simulink model "IARC_Nonlinear_Sensors"  (R2018a)
settings: Solver=ode1  StartTime=0.0  StopTime=20  FixedStep=T  RelTol=1e-3  EnableMultiTasking=on
undefined symbols (not defined in the file): A_1df, A_2df, alpha3, alpha_rp, alpha_x, alpha_z, an1, an1_v, an2, an3, bn1, bn1_v, bn2, bn3, dc_M_x, delta3, Epsilon3, F, g, Gamma1, Gamma2, Gamma3, Gamma4, gamma4_0, gamma_d_x, gamma_rp_0, gamma_x_0, gamma_z_0, Gammax, I, I_add, I_add_time, Jx, Jy, Jyaw, K, k1, k10, k11, k12, k2, k3, k4, k5, k6, k7, k8, k9, Ky, L, Light, LIMIT_CMD_PITCH, LIMIT_CMD_ROLL, LIMIT_CMD_xy, LIMIT_uCMD_HEIGHT, m, m_add, m_add_time, magnitude, MIL ... (+67)
libraries: simulink x131, simulink_extras x5, UAV_Control x4, aerolibwind2 x1
(part 5 of 6)

== system IARC_Nonlinear_Sensors/ARC Controller/Position Control/Coupling/Warm Up+Sat/Warm Up ==
  u : Inport
  z : Inport  Port=2
  z_des : Inport  Port=3
  " rising " : simulink/Logic and Bit Operations/Compare To Constant  Commented=on  relop=>  const=0  OutDataTypeStr=boolean
  4 : Scope  Commented=on
  6 : Scope  Commented=on
  Compare To Constant1 : simulink/Logic and Bit Operations/Compare To Constant  relop=>=  const=Zg+2/100  OutDataTypeStr=boolean
  Compare To Constant2 : simulink/Logic and Bit Operations/Compare To Constant  relop=>=  const=Zg+2/1000  OutDataTypeStr=boolean
  Data Type Conversion : DataTypeConversion
  Data Type Conversion1 : DataTypeConversion
  Data Type Conversion2 : DataTypeConversion
  InitializationDelay : Subsystem  AncestorBlock=UAV_Control/InitializationDelay  mask(InitializationDelay){t0=t0}
      mask prompts: t0 "Initialization delay:"
      mask help: Applays a delay before passing the first signal.
      mask Help: Applays a delay (t0) before passing the first signal
      mask Display:
      | port_label('input',1,'u','texmode','on')
      | port_label('output',1,'y','texmode','on')
  Is U capable of lifting the quad? : simulink/Logic and Bit Operations/Compare To Constant  relop=>=  const=0.69*m*g  OutDataTypeStr=boolean
  Is the quad commanded to move of the ground? : simulink/Logic and Bit Operations/Compare To Constant  relop=>  const=Zg  OutDataTypeStr=boolean
  Is the quad commanded to move of the ground?1 : simulink/Logic and Bit Operations/Compare To Constant  Commented=on  relop=<=  const=Zg+2/100  OutDataTypeStr=boolean
  Is the quad is commanded to move of the ground?2 : simulink/Logic and Bit Operations/Compare To Constant  relop===  const=Zg  OutDataTypeStr=boolean
  Logical Operator : Logic  AllPortsSameDT=off  OutDataTypeStr=boolean
  Logical Operator1 : Logic  Commented=on  AllPortsSameDT=off  OutDataTypeStr=boolean
  Mux6 : Mux  Commented=on  Inputs=3
  Rate Limiter : RateLimiter  RisingSlewLimit=m*g/2  FallingSlewLimit=-m*g/10  SampleTimeMode=inherited
  Saturation : Saturate  UpperLimit=Sat  LowerLimit=0.001
  Switch : Switch  Criteria=u2 > Threshold  Threshold=0.5
  Triggered Subsystem : Subsystem  TreatAsAtomicUnit=on
  z_ddot : simulink/Discrete/Discrete Derivative  Commented=on  gainval=1.0  ICPrevScaledInput=0.0  InputProcessing=Inherited  OutMin=[]  OutMax=[]  OutDataType=fixdt(1, 16)  OutScaling=2^-10  DoSatur=off
  z_des1 : InportShadow  Port=3
  y : Outport
  Adapt_M : Outport  Port=2
  Adapt_J : Outport  Port=3
  Land : Outport  Port=4
  takeoff2 : Outport  Port=5
  wires:
  u/1 -> Mux6/1, Switch/1, InitializationDelay/1(u)
  InitializationDelay/1(y) -> Rate Limiter/1
  Rate Limiter/1 -> Saturation/1
  Logical Operator/1 -> Data Type Conversion/1
  Data Type Conversion/1 -> Triggered Subsystem/Trigger, Triggered Subsystem/1(" ")
  Triggered Subsystem/1("  ") -> 4/1, Switch/2, Adapt_M/1
  Mux6/1 -> 6/1
  Switch/1 -> Mux6/3, y/1
  z/1 -> Compare To Constant2/1, z_ddot/1, Is the quad commanded to move of the ground?1/1, Compare To Constant1/1
  Compare To Constant1/1 -> Data Type Conversion1/1
  Data Type Conversion1/1 -> Adapt_J/1
  Is U capable of lifting the quad?/1 -> Logical Operator/1
  Is the quad commanded to move of the ground?/1 -> Logical Operator/2
  z_des/1 -> Is the quad commanded to move of the ground?/1
  Saturation/1 -> Mux6/2, Switch/3, Is U capable of lifting the quad?/1
  z_des1/1 -> Is the quad is commanded to move of the ground?2/1
  Is the quad is commanded to move of the ground?2/1 -> Land/1
  Compare To Constant2/1 -> Data Type Conversion2/1
  Data Type Conversion2/1 -> takeoff2/1
  Is the quad commanded to move of the ground?1/1 -> Logical Operator1/1
  z_ddot/1 -> " rising "/1
  " rising "/1 -> Logical Operator1/2
  Logical Operator1/1 -> ?

== system IARC_Nonlinear_Sensors/ARC Controller/Position Control/X control/Adaptation Law_X/  ==
  1 : Scope
  Constant4 : Constant  Value=m
  Divide : Product  Inputs=*/
  Selector : Selector  InputPortWidth=3  IndexOptions=Index vector (dialog)  Indices=1  OutputSizes=1
  Sum : Sum  Inputs=|++
  m_add : Step  Time=m_add_time  After=m_add(1,1)  SampleTime=0
  Out1 : Outport
  wires:
  [Fd] -> Selector/1
  Divide/1 -> 1/1, Out1/1
  Sum/1 -> Divide/2
  Constant4/1 -> Sum/1
  m_add/1 -> Sum/2
  Selector/1 -> Divide/1

== system IARC_Nonlinear_Sensors/ARC Controller/Position Control/X control/Adaptation Law_X/IARC, Physical Model Based Parameter Estimation (69)_X ==
  f(x) : Inport
  Phi : Inport  Port=2
  Adapt : Inport  Port=3
  Adapt1 : InportShadow  Port=3
  Constant2 : Constant  Value=Norm_ON
  Discontinuous_Proj_(49) : Subsystem
  Display : Display  Commented=on
  Divide : Product  Inputs=*/
  Epsilon : Subsystem
  Filter : Subsystem
  Gamma : Subsystem
  Switch1 : Switch  Threshold=0.5
  Theta_hat_dot : Product  Inputs=3  Multiplication=Matrix(*)
  den : Scope  Commented=on
  "epsilon  " : Scope  Commented=on
  gamma : Scope  Commented=on
  theta dot : Scope  Commented=on
  theta hat : Scope  Commented=on
  Theta_hat : Outport
  wires:
  Epsilon/1(Epsilon) -> Theta_hat_dot/3, "epsilon  "/1  "predicted output error"
  Discontinuous_Proj_(49)/1(Theta) -> theta hat/1, Theta_hat/1, Epsilon/3(Theta_hat)
  Filter/1(f(x)_f) -> Epsilon/1(f(x)_f_dot)
  Phi/1 -> Filter/2("Phi ")
  f(x)/1 -> Filter/1(f(x))
  Theta_hat_dot/1 -> Discontinuous_Proj_(49)/1(Theta_dot), theta dot/1
  Constant2/1 -> Switch1/2
  Gamma/1(" gamma") -> Display/1, gamma/1, Switch1/3, Divide/1
  Switch1/1 -> Theta_hat_dot/1
  Divide/1 -> Switch1/1
  Gamma/2(" 1+nu.Phi.G.Phi") -> den/1, Divide/2
  Filter/2(Phi_f) -> Epsilon/2(Phi_f), Gamma/1(Phi_f), Theta_hat_dot/2
  Adapt/1 -> Gamma/2(Adapt)
  Adapt1/1 -> Discontinuous_Proj_(49)/2(Adapt)

== system IARC_Nonlinear_Sensors/ARC Controller/Position Control/X control/Adaptation Law_X/Integral Type Adaptation Law Discontinuous Projection1 ==
  Phi : Inport
  error : Inport  Port=2
  {1..5} (5 alike) : Scope  Commented=on
  Constant : Constant  Value=gamma
  Constant2 : Constant  Value=Adaptation_ON
  Discontinuous Projection : Integrator  InitialCondition=theta0  LimitOutput=on  UpperSaturationLimit=theta_max  LowerSaturationLimit=theta_min
  Discontinuous Projection1 : Integrator  Commented=on  InitialCondition=theta0  UpperSaturationLimit=theta_max  LowerSaturationLimit=theta_min
  Gain : Gain  Commented=on  Gain=PSI
  InitializationDelay : Subsystem  AncestorBlock=UAV_Control/InitializationDelay  mask(InitializationDelay){t0=t1}
      mask prompts: t0 "Initialization delay:"
      mask help: Applays a delay before passing the first signal.
      mask Help: Applays a delay (t0) before passing the first signal
      mask Display:
      | port_label('input',1,'u','texmode','on')
      | port_label('output',1,'y','texmode','on')
  Product1 : Product  Inputs=3  Multiplication=Matrix(*)
  Saturation : Saturate  Commented=on  UpperLimit=theta_max  LowerLimit=theta_min
  Sum : Sum  Commented=on  Inputs=|++
  Sum1 : Sum  Commented=on  Inputs=-|+
  Switch1 : Switch  Criteria=u2 ~= 0
  real : Constant  Value=theta
  theta_est : Outport
  wires:
  Constant/1 -> Product1/1
  error/1 -> 2/1, Product1/3
  real/1 -> Switch1/3
  Constant2/1 -> Switch1/2
  Product1/1 -> InitializationDelay/1(u)
  Phi/1 -> 3/1, Product1/2
  InitializationDelay/1(y) -> Discontinuous Projection/1, 4/1, Sum/1
  Switch1/1 -> theta_est/1
  Sum/1 -> Discontinuous Projection1/1
  Discontinuous Projection1/1 -> Sum1/1, Saturation/1
  Sum1/1 -> Gain/1
  Gain/1 -> Sum/2
  Saturation/1 -> 1/1, Sum1/2
  Discontinuous Projection/1 -> 5/1, Switch1/1

== system IARC_Nonlinear_Sensors/ARC Controller/Position Control/X control/Adaptation Law_X/Subsystem1 ==
  u : Inport
  6 : Scope
  Constant4 : Constant  Value=m
  Divide : Product  Inputs=**
  Sum : Sum  Inputs=|++
  m_add : Step  Time=m_add_time  After=m_add  SampleTime=0
  y : Outport
  wires:
  u/1 -> Divide/1
  m_add/1 -> Sum/2
  Divide/1 -> y/1
  Sum/1 -> Divide/2, 6/1
  Constant4/1 -> Sum/1

== system IARC_Nonlinear_Sensors/ARC Controller/Position Control/Y control/Adaptation Law_Y/  ==
  1 : Scope
  Constant4 : Constant  Value=m
  Divide : Product  Inputs=*/
  Selector : Selector  InputPortWidth=3  IndexOptions=Index vector (dialog)  Indices=1  OutputSizes=1
  Sum : Sum  Inputs=|++
  m_add : Step  Time=m_add_time  After=m_add(1,1)  SampleTime=0
  Out1 : Outport
  wires:
  [Fd] -> Selector/1
  Divide/1 -> 1/1, Out1/1
  Sum/1 -> Divide/2
  Constant4/1 -> Sum/1
  m_add/1 -> Sum/2
  Selector/1 -> Divide/1

== system IARC_Nonlinear_Sensors/ARC Controller/Position Control/Y control/Adaptation Law_Y/IARC, Physical Model Based Parameter Estimation (69)_X ==
  f(x) : Inport
  Phi : Inport  Port=2
  Adapt : Inport  Port=3
  Adapt1 : InportShadow  Port=3
  Constant2 : Constant  Value=Norm_ON
  Discontinuous_Proj_(49) : Subsystem
  Display : Display  Commented=on
  Divide : Product  Inputs=*/
  Epsilon : Subsystem
  Filter : Subsystem
  Gamma : Subsystem
  Switch1 : Switch  Threshold=0.5
  Theta_hat_dot : Product  Inputs=3  Multiplication=Matrix(*)
  "epsilon  " : Scope  Commented=on
  gamma : Scope  Commented=on
  theta dot : Scope  Commented=on
  theta hat : Scope  Commented=on
  Theta_hat : Outport
  wires:
  Epsilon/1(Epsilon) -> Theta_hat_dot/3, "epsilon  "/1  "predicted output error"
  Discontinuous_Proj_(49)/1(Theta) -> theta hat/1, Theta_hat/1, Epsilon/3(Theta_hat)
  Filter/1(f(x)_f) -> Epsilon/1(f(x)_f_dot)
  Phi/1 -> Filter/2("Phi ")
  f(x)/1 -> Filter/1(f(x))
  Theta_hat_dot/1 -> Discontinuous_Proj_(49)/1(Theta_dot), theta dot/1
  Constant2/1 -> Switch1/2
  Gamma/1(" gamma") -> Display/1, gamma/1, Switch1/3, Divide/1
  Switch1/1 -> Theta_hat_dot/1
  Divide/1 -> Switch1/1
  Gamma/2(" 1+nu.Phi.G.Phi") -> Divide/2
  Filter/2(Phi_f) -> Epsilon/2(Phi_f), Gamma/1(Phi_f), Theta_hat_dot/2
  Adapt/1 -> Gamma/2(Adapt)
  Adapt1/1 -> Discontinuous_Proj_(49)/2(Adapt)

== system IARC_Nonlinear_Sensors/ARC Controller/Position Control/Y control/Adaptation Law_Y/Integral Type Adaptation Law Discontinuous Projection1 ==
  Phi : Inport
  error : Inport  Port=2
  {1..5} (5 alike) : Scope  Commented=on
  Constant : Constant  Value=gamma
  Constant2 : Constant  Value=Adaptation_ON
  Discontinuous Projection : Integrator  InitialCondition=theta0  LimitOutput=on  UpperSaturationLimit=theta_max  LowerSaturationLimit=theta_min
  Discontinuous Projection1 : Integrator  Commented=on  InitialCondition=theta0  UpperSaturationLimit=theta_max  LowerSaturationLimit=theta_min
  Gain : Gain  Commented=on  Gain=PSI
  InitializationDelay : Subsystem  AncestorBlock=UAV_Control/InitializationDelay  mask(InitializationDelay){t0=t1}
      mask prompts: t0 "Initialization delay:"
      mask help: Applays a delay before passing the first signal.
      mask Help: Applays a delay (t0) before passing the first signal
      mask Display:
      | port_label('input',1,'u','texmode','on')
      | port_label('output',1,'y','texmode','on')
  Product1 : Product  Inputs=3  Multiplication=Matrix(*)
  Saturation : Saturate  Commented=on  UpperLimit=theta_max  LowerLimit=theta_min
  Sum : Sum  Commented=on  Inputs=|++
  Sum1 : Sum  Commented=on  Inputs=-|+
  Switch1 : Switch  Criteria=u2 ~= 0
  real : Constant  Value=theta
  theta_est : Outport
  wires:
  Constant/1 -> Product1/1
  error/1 -> 2/1, Product1/3
  real/1 -> Switch1/3
  Constant2/1 -> Switch1/2
  Product1/1 -> InitializationDelay/1(u)
  Phi/1 -> 3/1, Product1/2
  InitializationDelay/1(y) -> Discontinuous Projection/1, 4/1, Sum/1
  Switch1/1 -> theta_est/1
  Sum/1 -> Discontinuous Projection1/1
  Discontinuous Projection1/1 -> Sum1/1, Saturation/1
  Sum1/1 -> Gain/1
  Gain/1 -> Sum/2
  Saturation/1 -> 1/1, Sum1/2
  Discontinuous Projection/1 -> 5/1, Switch1/1

== system IARC_Nonlinear_Sensors/ARC Controller/Position Control/Y control/Adaptation Law_Y/Subsystem1 ==
  u : Inport
  6 : Scope
  Constant4 : Constant  Value=m
  Divide : Product  Inputs=**
  Sum : Sum  Inputs=|++
  m_add : Step  Time=m_add_time  After=m_add  SampleTime=0
  y : Outport
  wires:
  u/1 -> Divide/1
  m_add/1 -> Sum/2
  Divide/1 -> y/1
  Sum/1 -> Divide/2, 6/1
  Constant4/1 -> Sum/1

== system IARC_Nonlinear_Sensors/ARC Controller/Position Control/Z control/Estimate theta = K//m/IARC, Physical Model Based Parameter Estimation (69) ==
  y : Inport
  Phi : Inport  Port=2
  Adapt1 : Inport  Port=3
  Adapt2 : InportShadow  Port=3
  Constant2 : Constant  Value=Norm_ON
  Discontinuous_Proj_(49) : Subsystem
  Display : Display  Commented=on
  Divide : Product  Inputs=*/
  Epsilon : Subsystem
  Filter : Subsystem
  Gamma : Subsystem
  Switch1 : Switch  Threshold=0.5
  Theta_hat_dot : Product  Inputs=3  Multiplication=Matrix(*)
  "epsilon  " : Scope  Commented=on
  gamma : Scope  Commented=on
  theta dot : Scope  Commented=on
  theta hat : Scope  Commented=on
  Theta_hat : Outport
  wires:
  Adapt1/1 -> Discontinuous_Proj_(49)/2(Adapt)
  Filter/2(Phi_f) -> Epsilon/2(Phi_f), Gamma/1(Phi_f), Theta_hat_dot/2
  Epsilon/1(Epsilon) -> "epsilon  "/1, Theta_hat_dot/3  "predicted output error"
  Discontinuous_Proj_(49)/1(Theta) -> Theta_hat/1, theta hat/1, Epsilon/3(Theta_hat)
  Filter/1(y_f) -> Epsilon/1(y_f)
  Phi/1 -> Filter/2("Phi ")
  y/1 -> Filter/1(y)
  Theta_hat_dot/1 -> Discontinuous_Proj_(49)/1(Theta_dot), theta dot/1
  Constant2/1 -> Switch1/2
  Gamma/1(" gamma") -> Display/1, gamma/1, Switch1/3, Divide/1
  Switch1/1 -> Theta_hat_dot/1
  Divide/1 -> Switch1/1
  Gamma/2(" 1+nu.Phi.G.Phi") -> Divide/2
  Adapt2/1 -> Gamma/2(Adapt)

== system IARC_Nonlinear_Sensors/ARC Controller/Position Control/Z control/Estimate theta = K//m/Integral Type Adaptation Law Discontinuous Projection ==
  Phi : Inport
  error : Inport  Port=2
  {1..5,11} (6 alike) : Scope  Commented=on
  Constant : Constant  Value=gamma
  Constant2 : Constant  Value=Adaptation_ON
  Discontinuous Projection : Integrator  InitialCondition=theta0  LimitOutput=on  UpperSaturationLimit=theta_max  LowerSaturationLimit=theta_min
  Discontinuous Projection1 : Integrator  Commented=on  InitialCondition=theta0  UpperSaturationLimit=theta_max  LowerSaturationLimit=theta_min
  Gain : Gain  Commented=on  Gain=PSI
  InitializationDelay : Subsystem  AncestorBlock=UAV_Control/InitializationDelay  mask(InitializationDelay){t0=t1}
      mask prompts: t0 "Initialization delay:"
      mask help: Applays a delay before passing the first signal.
      mask Help: Applays a delay (t0) before passing the first signal
      mask Display:
      | port_label('input',1,'u','texmode','on')
      | port_label('output',1,'y','texmode','on')
  Product1 : Product  Inputs=3  Multiplication=Matrix(*)
  Saturation : Saturate  Commented=on  UpperLimit=theta_max  LowerLimit=theta_min
  Sum : Sum  Commented=on  Inputs=|++
  Sum1 : Sum  Commented=on  Inputs=-|+
  Switch1 : Switch  Criteria=u2 ~= 0
  real : Constant  Value=theta
  theta_est : Outport
  wires:
  Constant/1 -> Product1/1
  error/1 -> 2/1, Product1/3
  real/1 -> Switch1/3
  Constant2/1 -> Switch1/2
  Product1/1 -> InitializationDelay/1(u)
  Phi/1 -> 3/1, Product1/2
  InitializationDelay/1(y) -> Discontinuous Projection/1, 4/1, Sum/1, 11/1
  Switch1/1 -> theta_est/1
  Sum/1 -> Discontinuous Projection1/1
  Discontinuous Projection1/1 -> Sum1/1, Saturation/1
  Sum1/1 -> Gain/1
  Gain/1 -> Sum/2
  Saturation/1 -> 1/1, Sum1/2
  Discontinuous Projection/1 -> 5/1, Switch1/1

== system IARC_Nonlinear_Sensors/ARC Controller/Position Control/Z control/Estimate theta = K//m/m ==
  Constant4 : Constant  Value=m
  Gain : Gain  Gain=K
  Math Function : Math  Operator=reciprocal  SaturateOnIntegerOverflow=on
  Step : Step  Time=m_add_time  After=m_add  SampleTime=0
  Sum : Sum  Inputs=|++
  Out1 : Outport
  wires:
  Constant4/1 -> Sum/1
  Step/1 -> Sum/2
  Math Function/1 -> Gain/1
  Gain/1 -> Out1/1
  Sum/1 -> Math Function/1

== system IARC_Nonlinear_Sensors/Sensors and Filters/Data processing/Estimate Position/Signal Conditioning - Sonar/FOH1 ==
  Input : Inport
  Bias : Bias  Bias=-Ts
  Clock : Clock
      settings: DisableCoverage=on
  Digital Clock : DigitalClock  DisableCoverage=on  SampleTime=Ts
  Gain : Gain  DisableCoverage=on  Gain=1/Ts  SaturateOnIntegerOverflow=on  OutDataTypeStr=Inherit: Same as input  ParamDataTypeStr=Inherit: Same as input
  Product : Product  RndMeth=Zero
  Rate Transition : RateTransition
  Rate Transition1 : RateTransition  OutPortSampleTime=T
  Rate Transition3 : RateTransition  OutPortSampleTime=T
  Rate Transition4 : RateTransition  OutPortSampleTime=Ts
  Rate Transition5 : RateTransition  OutPortSampleTime=T
  Scope : Scope
  Scope1 : Scope
  Sum : Sum  DisableCoverage=on  Inputs=|+-  SaturateOnIntegerOverflow=on  InputSameDT=on  OutDataTypeStr=Inherit: Same as first input
  Sum2 : Sum  DisableCoverage=on  Inputs=|+-  SaturateOnIntegerOverflow=on  InputSameDT=on  OutDataTypeStr=Inherit: Same as first input
  Unit Delay : UnitDelay  DisableCoverage=on  SampleTime=Ts
  s : Sum  Inputs=++|  SaturateOnIntegerOverflow=on  InputSameDT=on  OutDataTypeStr=Inherit: Same as first input
  Output : Outport
  wires:
  Rate Transition4/1 -> Unit Delay/1, Sum/1
  Input/1 -> Rate Transition4/1, Rate Transition5/1
  Unit Delay/1 -> Sum/2
  Rate Transition1/1 -> Product/1, Scope1/1
  Product/1 -> s/2
  Rate Transition3/1 -> Product/2, Scope/1
  Sum/1 -> Rate Transition1/1
  Bias/1 -> Sum2/1
  Clock/1 -> Bias/1
  Rate Transition/1 -> Sum2/2
  s/1 -> Output/1
  Rate Transition5/1 -> s/1
  Gain/1 -> Rate Transition3/1
  Digital Clock/1 -> Rate Transition/1
  Sum2/1 -> Gain/1

== system IARC_Nonlinear_Sensors/Sensors and Filters/Data processing/Estimate Position/Signal Conditioning - Sonar/Sampler ==
  In1 : Inport
  Derivative : Derivative
  Digital Clock : DigitalClock  DisableCoverage=on  SampleTime=0.1
  Rate Transition : RateTransition
  Triggered Subsystem : Subsystem  TreatAsAtomicUnit=on
  Out1 : Outport
  wires:
  Derivative/1 -> Triggered Subsystem/Trigger
  Rate Transition/1 -> Derivative/1
  Digital Clock/1 -> Rate Transition/1
  In1/1 -> Triggered Subsystem/1(In1)
  Triggered Subsystem/1(Out1) -> Out1/1

== system IARC_Nonlinear_Sensors/ARC Controller/Attitutde Control/Subsystem/f/d(T)//d(phi)/Subsystem ==
  In1 : Inport
  In2 : Inport  Port=2
  In3 : Inport  Port=3
  In4 : Inport  Port=4
  In5 : Inport  Port=5
  In6 : Inport  Port=6
  In7 : Inport  Port=7
  In8 : Inport  Port=8
  In9 : Inport  Port=9
  Matrix Concatenate : Concatenate  NumInputs=3  Mode=Multidimensional array  ConcatenateDimension=2
  Mux : Mux  Inputs=3
  Mux1 : Mux  Inputs=3
  Mux2 : Mux  Inputs=3
  Reshape : Reshape  OutputDimensionality=Column vector (2-D)
  Reshape1 : Reshape  OutputDimensionality=Column vector (2-D)
  Reshape2 : Reshape  OutputDimensionality=Column vector (2-D)
  Out1 : Outport
  wires:
  Reshape1/1 -> Matrix Concatenate/2
  Mux1/1 -> Reshape1/1
  Reshape/1 -> Matrix Concatenate/1
  Reshape2/1 -> Matrix Concatenate/3
  Matrix Concatenate/1 -> Out1/1
  Mux2/1 -> Reshape2/1
  Mux/1 -> Reshape/1
  In1/1 -> Mux/1
  In2/1 -> Mux/2
  In3/1 -> Mux/3
  In4/1 -> Mux1/1
  In5/1 -> Mux1/2
  In6/1 -> Mux1/3
  In7/1 -> Mux2/1
  In8/1 -> Mux2/2
  In9/1 -> Mux2/3

== system IARC_Nonlinear_Sensors/ARC Controller/Attitutde Control/Subsystem/f/d(T)//d(theta)/Subsystem ==
  In1 : Inport
  In2 : Inport  Port=2
  In3 : Inport  Port=3
  In4 : Inport  Port=4
  In5 : Inport  Port=5
  In6 : Inport  Port=6
  In7 : Inport  Port=7
  In8 : Inport  Port=8
  In9 : Inport  Port=9
  Matrix Concatenate : Concatenate  NumInputs=3  Mode=Multidimensional array  ConcatenateDimension=2
  Mux : Mux  Inputs=3
  Mux1 : Mux  Inputs=3
  Mux2 : Mux  Inputs=3
  Reshape : Reshape  OutputDimensionality=Column vector (2-D)
  Reshape1 : Reshape  OutputDimensionality=Column vector (2-D)
  Reshape2 : Reshape  OutputDimensionality=Column vector (2-D)
  Out1 : Outport
  wires:
  In9/1 -> Mux2/3
  In8/1 -> Mux2/2
  In7/1 -> Mux2/1
  In6/1 -> Mux1/3
  In5/1 -> Mux1/2
  In4/1 -> Mux1/1
  In3/1 -> Mux/3
  In2/1 -> Mux/2
  In1/1 -> Mux/1
  Mux/1 -> Reshape/1
  Mux2/1 -> Reshape2/1
  Matrix Concatenate/1 -> Out1/1
  Reshape2/1 -> Matrix Concatenate/3
  Reshape/1 -> Matrix Concatenate/1
  Mux1/1 -> Reshape1/1
  Reshape1/1 -> Matrix Concatenate/2

== system IARC_Nonlinear_Sensors/ARC Controller/Attitutde Control/Yaw control/Subsystem/IARC, Physical Model Based Parameter Estimation (69)_Yaw/Discontinuous_Proj_(49) ==
  Theta_dot : Inport
  Adapt : Inport  Port=2
  Integrator2 : Integrator  InitialCondition=theta_0  LimitOutput=on  UpperSaturationLimit=theta_max  LowerSaturationLimit=theta_min
  Product : Product
  Saturation : Saturate  UpperLimit=Theta_dot_M  LowerLimit=-Theta_dot_M
  Theta : Outport
  wires:
  Integrator2/1 -> Theta/1
  Product/1 -> Saturation/1
  Saturation/1 -> Integrator2/1
  Adapt/1 -> Product/2
  Theta_dot/1 -> Product/1

== system IARC_Nonlinear_Sensors/ARC Controller/Attitutde Control/Yaw control/Subsystem/IARC, Physical Model Based Parameter Estimation (69)_Yaw/Epsilon ==
  f(x)_f_dot : Inport
  Phi_f : Inport  Port=2
  Theta_hat : Inport  Port=3
  Math Function : Math  Operator=transpose  SaturateOnIntegerOverflow=on
  Mux1 : Mux  Inputs=3
  Product1 : Product  Multiplication=Matrix(*)
  Subtract : Sum  Inputs=+-
  "epsilon  " : Scope
  Epsilon : Outport
  wires:
  f(x)_f_dot/1 -> Mux1/2, Subtract/1  "Yp"
  Product1/1 -> Mux1/3, Subtract/2  "Yp_hat"
  Phi_f/1 -> Math Function/1
  Theta_hat/1 -> Product1/2
  Math Function/1 -> Product1/1
  Subtract/1 -> Mux1/1, Epsilon/1
  Mux1/1 -> "epsilon  "/1

== system IARC_Nonlinear_Sensors/ARC Controller/Attitutde Control/Yaw control/Subsystem/IARC, Physical Model Based Parameter Estimation (69)_Yaw/Filter ==
  f(x) : Inport
  "Phi " : Inport  Port=2
  Demux : Demux  Outputs=2
  Mux1 : Mux  Commented=on  Inputs=2
  Mux2 : Mux  Commented=on  Inputs=2
  Mux3 : Mux  Inputs=2
  filter : TransferFcn  Denominator=[Tau 1]
  "filter " : TransferFcn  Denominator=[Tau 1]
  filter1 : TransferFcn  Denominator=[Tau 1]
  gamma : Scope  Commented=on
  gamma1 : Scope  Commented=on
  f(x)_f : Outport
  Phi_f : Outport  Port=2
  wires:
  "Phi "/1 -> Demux/1
  "filter "/1 -> f(x)_f/1, Mux1/2
  f(x)/1 -> Mux1/1, "filter "/1
  Mux1/1 -> gamma/1
  Demux/1 -> Mux2/1, filter/1
  Mux2/1 -> gamma1/1
  filter/1 -> Mux2/2, Mux3/1
  Demux/2 -> filter1/1
  filter1/1 -> Mux3/2
  Mux3/1 -> Phi_f/1

== system IARC_Nonlinear_Sensors/ARC Controller/Attitutde Control/Yaw control/Subsystem/IARC, Physical Model Based Parameter Estimation (69)_Yaw/Gamma ==
  Phi_f : Inport
  Adapt : Inport  Port=2
  " " : Constant  Value=diag(0,0)
  Gamma_dot : Subsystem
  InitializationDelay : Subsystem  AncestorBlock=UAV_Control/InitializationDelay  mask(InitializationDelay){t0=t1}
      mask prompts: t0 "Initialization delay:"
      mask help: Applays a delay before passing the first signal.
      mask Help: Applays a delay (t0) before passing the first signal
      mask Display:
      | port_label('input',1,'u','texmode','on')
      | port_label('output',1,'y','texmode','on')
  Product : Product
  Switch : Switch  Criteria=u2 > Threshold
  "gamma " : Integrator  InitialCondition=gamma0  LimitOutput=on  UpperSaturationLimit=Rho_M  LowerSaturationLimit=Rho_L
  vDv : Subsystem
  " gamma" : Outport
  " 1+nu.Phi.G.Phi" : Outport  Port=2
  wires:
  "gamma "/1 -> [gamma], " gamma"/1
  " "/1 -> Switch/1
  vDv/1(Out1) -> Switch/2
  Phi_f/1 -> Gamma_dot/1(Phi_f)
  Gamma_dot/1(gamma_dot) -> InitializationDelay/1(u)
  [gamma] -> Gamma_dot/2(Gamma)
  Gamma_dot/2(" 1+nu.Phi.G.Phi") -> " 1+nu.Phi.G.Phi"/1
  Product/1 -> "gamma "/1, Switch/3, vDv/1(In1)
  InitializationDelay/1(y) -> Product/1
  Adapt/1 -> Product/2

== system IARC_Nonlinear_Sensors/ARC Controller/Attitutde Control/pitch control/Adaptation Law_X/IARC, Physical Model Based Parameter Estimation (69)_pitch (theta)/Discontinuous_Proj_(49) ==
  Theta_dot : Inport
  Adapt : Inport  Port=2
  Integrator2 : Integrator  InitialCondition=theta_0  LimitOutput=on  UpperSaturationLimit=theta_max  LowerSaturationLimit=theta_min
  Product : Product
  Saturation : Saturate  UpperLimit=Theta_dot_M  LowerLimit=-Theta_dot_M
  Theta : Outport
  wires:
  Integrator2/1 -> Theta/1
  Product/1 -> Saturation/1
  Saturation/1 -> Integrator2/1
  Adapt/1 -> Product/2
  Theta_dot/1 -> Product/1

== system IARC_Nonlinear_Sensors/ARC Controller/Attitutde Control/pitch control/Adaptation Law_X/IARC, Physical Model Based Parameter Estimation (69)_pitch (theta)/Epsilon ==
  f(x)_f_dot : Inport
  Phi_f : Inport  Port=2
  Theta_hat : Inport  Port=3
  Math Function : Math  Operator=transpose  SaturateOnIntegerOverflow=on
  Mux1 : Mux  Inputs=3
  Product1 : Product  Multiplication=Matrix(*)
  Subtract : Sum  Inputs=+-
  "epsilon  " : Scope
  Epsilon : Outport
  wires:
  f(x)_f_dot/1 -> Mux1/2, Subtract/1  "Yp"
  Subtract/1 -> Mux1/1, Epsilon/1
  Product1/1 -> Subtract/2, Mux1/3  "Yp_hat"
  Phi_f/1 -> Math Function/1
  Theta_hat/1 -> Product1/2
  Math Function/1 -> Product1/1
  Mux1/1 -> "epsilon  "/1

== system IARC_Nonlinear_Sensors/ARC Controller/Attitutde Control/pitch control/Adaptation Law_X/IARC, Physical Model Based Parameter Estimation (69)_pitch (theta)/Filter ==
  f(x) : Inport
  "Phi " : Inport  Port=2
  Demux : Demux  Outputs=2
  Mux1 : Mux  Commented=on  Inputs=2
  Mux2 : Mux  Commented=on  Inputs=2
  Mux3 : Mux  Inputs=2
  filter : TransferFcn  Denominator=[Tau 1]
  "filter " : TransferFcn  Denominator=[Tau 1]
  filter1 : TransferFcn  Denominator=[Tau 1]
  gamma : Scope  Commented=on
  u_f : Scope  Commented=on
  f(x)_f : Outport
  Phi_f : Outport  Port=2
  wires:
  Mux3/1 -> Phi_f/1
  "filter "/1 -> f(x)_f/1, Mux1/2
  f(x)/1 -> Mux1/1, "filter "/1
  Mux1/1 -> gamma/1
  Demux/1 -> Mux2/1, filter/1
  Mux2/1 -> u_f/1
  filter/1 -> Mux2/2, Mux3/1
  "Phi "/1 -> Demux/1
  Demux/2 -> filter1/1
  filter1/1 -> Mux3/2

== system IARC_Nonlinear_Sensors/ARC Controller/Attitutde Control/pitch control/Adaptation Law_X/IARC, Physical Model Based Parameter Estimation (69)_pitch (theta)/Gamma ==
  Phi_f : Inport
  Adapt : Inport  Port=2
  " " : Constant  Value=diag(0,0)
  Gamma_dot : Subsystem
  InitializationDelay : Subsystem  AncestorBlock=UAV_Control/InitializationDelay  mask(InitializationDelay){t0=t1}
      mask prompts: t0 "Initialization delay:"
      mask help: Applays a delay before passing the first signal.
      mask Help: Applays a delay (t0) before passing the first signal
      mask Display:
      | port_label('input',1,'u','texmode','on')
      | port_label('output',1,'y','texmode','on')
  Product : Product
  Scope{,1..3} (4 alike) : Scope  Commented=on
  Switch : Switch  Criteria=u2 > Threshold
  "gamma " : Integrator  InitialCondition=gamma0  LimitOutput=on  UpperSaturationLimit=Rho_M  LowerSaturationLimit=Rho_L
  vDv : Subsystem
  " gamma" : Outport
  " 1+nu.Phi.G.Phi" : Outport  Port=2
  wires:
  "gamma "/1 -> Scope3/1, [gamma], " gamma"/1
  " "/1 -> Switch/1
  vDv/1(Out1) -> Scope/1, Switch/2
  Phi_f/1 -> Gamma_dot/1(Phi_f)
  Gamma_dot/1(gamma_dot) -> Scope2/1, InitializationDelay/1(u)
  [gamma] -> Gamma_dot/2(Gamma)
  Gamma_dot/2(" 1+nu.Phi.G.Phi") -> " 1+nu.Phi.G.Phi"/1
  Product/1 -> "gamma "/1, Switch/3, vDv/1(In1)
  Switch/1 -> Scope1/1
  InitializationDelay/1(y) -> Product/1
  Adapt/1 -> Product/2

== system IARC_Nonlinear_Sensors/ARC Controller/Attitutde Control/roll control/Adaptation Law_Y/IARC, Physical Model Based Parameter Estimation (69)_roll (phi)/Discontinuous_Proj_(49) ==
  Theta_dot : Inport
  Adapt : Inport  Port=2
  Integrator2 : Integrator  InitialCondition=theta_0  LimitOutput=on  UpperSaturationLimit=theta_max  LowerSaturationLimit=theta_min
  Product : Product
  Saturation : Saturate  UpperLimit=Theta_dot_M  LowerLimit=-Theta_dot_M
  theta dot : Scope
  Theta : Outport
  wires:
  Integrator2/1 -> Theta/1
  Product/1 -> Saturation/1
  Saturation/1 -> theta dot/1, Integrator2/1
  Adapt/1 -> Product/2
  Theta_dot/1 -> Product/1

== system IARC_Nonlinear_Sensors/ARC Controller/Attitutde Control/roll control/Adaptation Law_Y/IARC, Physical Model Based Parameter Estimation (69)_roll (phi)/Epsilon ==
  f(x)_f_dot : Inport
  Phi_f : Inport  Port=2
  Theta_hat : Inport  Port=3
  Math Function : Math  Operator=transpose  SaturateOnIntegerOverflow=on
  Mux1 : Mux  Inputs=3
  Product1 : Product  Multiplication=Matrix(*)
  Subtract : Sum  Inputs=+-
  "epsilon  " : Scope
  Epsilon : Outport
  wires:
  f(x)_f_dot/1 -> Mux1/2, Subtract/1  "Yp"
  Subtract/1 -> Mux1/1, Epsilon/1
  Product1/1 -> Subtract/2, Mux1/3  "Yp_hat"
  Phi_f/1 -> Math Function/1
  Theta_hat/1 -> Product1/2
  Math Function/1 -> Product1/1
  Mux1/1 -> "epsilon  "/1

== system IARC_Nonlinear_Sensors/ARC Controller/Attitutde Control/roll control/Adaptation Law_Y/IARC, Physical Model Based Parameter Estimation (69)_roll (phi)/Filter ==
  f(x) : Inport
  "Phi " : Inport  Port=2
  Demux : Demux  Outputs=2
  Mux1 : Mux  Commented=on  Inputs=2
  Mux2 : Mux  Commented=on  Inputs=2
  Mux3 : Mux  Inputs=2
  filter : TransferFcn  Denominator=[Tau 1]
  "filter " : TransferFcn  Denominator=[Tau 1]
  filter1 : TransferFcn  Denominator=[Tau 1]
  gamma : Scope  Commented=on
  u_f : Scope  Commented=on
  f(x)_f : Outport
  Phi_f : Outport  Port=2
  wires:
  Mux3/1 -> Phi_f/1
  "filter "/1 -> f(x)_f/1, Mux1/2
  f(x)/1 -> Mux1/1, "filter "/1
  Mux1/1 -> gamma/1
  Demux/1 -> Mux2/1, filter/1
  Mux2/1 -> u_f/1
  filter/1 -> Mux2/2, Mux3/1
  "Phi "/1 -> Demux/1
  Demux/2 -> filter1/1
  filter1/1 -> Mux3/2

== system IARC_Nonlinear_Sensors/ARC Controller/Attitutde Control/roll control/Adaptation Law_Y/IARC, Physical Model Based Parameter Estimation (69)_roll (phi)/Gamma ==
  Phi_f : Inport
  Adapt : Inport  Port=2
  " " : Constant  Value=diag(0,0)
  Gamma_dot : Subsystem
  InitializationDelay : Subsystem  AncestorBlock=UAV_Control/InitializationDelay  mask(InitializationDelay){t0=t1}
      mask prompts: t0 "Initialization delay:"
      mask help: Applays a delay before passing the first signal.
      mask Help: Applays a delay (t0) before passing the first signal
      mask Display:
      | port_label('input',1,'u','texmode','on')
      | port_label('output',1,'y','texmode','on')
  Product : Product
  Scope{,1..3} (4 alike) : Scope  Commented=on
  Switch : Switch  Criteria=u2 > Threshold
  "gamma " : Integrator  InitialCondition=gamma0  LimitOutput=on  UpperSaturationLimit=Rho_M  LowerSaturationLimit=Rho_L
  vDv : Subsystem
  " gamma" : Outport
  " 1+nu.Phi.G.Phi" : Outport  Port=2
  wires:
  "gamma "/1 -> Scope3/1, [gamma], " gamma"/1
  " "/1 -> Switch/1
  vDv/1(Out1) -> Scope/1, Switch/2
  Phi_f/1 -> Gamma_dot/1(Phi_f)
  Gamma_dot/1(gamma_dot) -> Scope2/1, InitializationDelay/1(u)
  [gamma] -> Gamma_dot/2(Gamma)
  Gamma_dot/2(" 1+nu.Phi.G.Phi") -> " 1+nu.Phi.G.Phi"/1
  Product/1 -> "gamma "/1, Switch/3, vDv/1(In1)
  Switch/1 -> Scope1/1
  InitializationDelay/1(y) -> Product/1
  Adapt/1 -> Product/2

== system IARC_Nonlinear_Sensors/ARC Controller/Attitutde Control/roll control/Adaptation Law_Y/Integral Type Adaptation Law Discontinuous Projection/InitializationDelay ==
  u : Inport
  Clock : Clock
  Compare To Constant2 : simulink/Logic and Bit Operations/Compare To Constant  relop=>=  const=t0  OutDataTypeStr=boolean
  Data Type Conversion : DataTypeConversion
  Product : Product
  y : Outport
  wires:
  u/1 -> Product/1
  Compare To Constant2/1 -> Data Type Conversion/1
  Clock/1 -> Compare To Constant2/1
  Data Type Conversion/1 -> Product/2
  Product/1 -> y/1

== system IARC_Nonlinear_Sensors/ARC Controller/Position Control/Coupling/Warm Up+Sat/Warm Up/InitializationDelay ==
  u : Inport
  Clock : Clock
  Compare To Constant2 : simulink/Logic and Bit Operations/Compare To Constant  relop=>=  const=t0  OutDataTypeStr=boolean
  Data Type Conversion : DataTypeConversion
  Product : Product
  y : Outport
  wires:
  u/1 -> Product/1
  Compare To Constant2/1 -> Data Type Conversion/1
  Clock/1 -> Compare To Constant2/1
  Data Type Conversion/1 -> Product/2
  Product/1 -> y/1

== system IARC_Nonlinear_Sensors/ARC Controller/Position Control/Coupling/Warm Up+Sat/Warm Up/Triggered Subsystem ==
  " " : Inport
  Trigger : TriggerPort  VariantControl=Variant
  "  " : Outport
  wires:
  " "/1 -> "  "/1

== system IARC_Nonlinear_Sensors/ARC Controller/Position Control/X control/Adaptation Law_X/IARC, Physical Model Based Parameter Estimation (69)_X/Discontinuous_Proj_(49) ==
  Theta_dot : Inport
  Adapt : Inport  Port=2
  Integrator1 : Integrator  InitialCondition=theta_0  UpperSaturationLimit=theta_max  LowerSaturationLimit=theta_min
  Integrator2 : Integrator  Commented=on  InitialCondition=theta_0  LimitOutput=on  UpperSaturationLimit=theta_max  LowerSaturationLimit=theta_min
  Product : Product
  Saturation : Saturate  UpperLimit=Theta_dot_M  LowerLimit=-Theta_dot_M
  Theta : Outport
  wires:
  Integrator1/1 -> Theta/1
  Product/1 -> Saturation/1
  Saturation/1 -> Integrator1/1
  Adapt/1 -> Product/2
  Theta_dot/1 -> Product/1

== system IARC_Nonlinear_Sensors/ARC Controller/Position Control/X control/Adaptation Law_X/IARC, Physical Model Based Parameter Estimation (69)_X/Epsilon ==
  f(x)_f_dot : Inport
  Phi_f : Inport  Port=2
  Theta_hat : Inport  Port=3
  Math Function : Math  Operator=transpose  SaturateOnIntegerOverflow=on
  Mux1 : Mux  Inputs=3
  Product1 : Product  Multiplication=Matrix(*)
  Subtract : Sum  Inputs=+-
  "epsilon  " : Scope
  Epsilon : Outport
  wires:
  f(x)_f_dot/1 -> Mux1/2, Subtract/1  "Yp"
  Product1/1 -> Mux1/3, Subtract/2  "Yp_hat"
  Phi_f/1 -> Math Function/1
  Theta_hat/1 -> Product1/2
  Math Function/1 -> Product1/1
  Subtract/1 -> Mux1/1, Epsilon/1
  Mux1/1 -> "epsilon  "/1

== system IARC_Nonlinear_Sensors/ARC Controller/Position Control/X control/Adaptation Law_X/IARC, Physical Model Based Parameter Estimation (69)_X/Filter ==
  f(x) : Inport
  "Phi " : Inport  Port=2
  Mux1 : Mux  Commented=on  Inputs=2
  Mux2 : Mux  Commented=on  Inputs=2
  filter : TransferFcn  Denominator=[Tau 1]
  "filter " : TransferFcn  Denominator=[Tau 1]
  gamma : Scope  Commented=on
  gamma1 : Scope  Commented=on
  f(x)_f : Outport
  Phi_f : Outport  Port=2
  wires:
  f(x)/1 -> "filter "/1, Mux1/1
  Mux1/1 -> gamma/1
  Mux2/1 -> gamma1/1
  "Phi "/1 -> filter/1, Mux2/1
  "filter "/1 -> f(x)_f/1, Mux1/2
  filter/1 -> Mux2/2, Phi_f/1

== system IARC_Nonlinear_Sensors/ARC Controller/Position Control/X control/Adaptation Law_X/IARC, Physical Model Based Parameter Estimation (69)_X/Gamma ==
  Phi_f : Inport
  Adapt : Inport  Port=2
  " " : Constant  Value=diag(0,0)
  Gamma_dot : Subsystem
  InitializationDelay : Subsystem  AncestorBlock=UAV_Control/InitializationDelay  mask(InitializationDelay){t0=t1}
      mask prompts: t0 "Initialization delay:"
      mask help: Applays a delay before passing the first signal.
      mask Help: Applays a delay (t0) before passing the first signal
      mask Display:
      | port_label('input',1,'u','texmode','on')
      | port_label('output',1,'y','texmode','on')
  Product : Product
  Scope{,1..3} (4 alike) : Scope  Commented=on
  Switch : Switch  Criteria=u2 > Threshold
  "gamma " : Integrator  InitialCondition=gamma0  LimitOutput=on  UpperSaturationLimit=Rho_M  LowerSaturationLimit=Rho_L
  vDv : Subsystem
  " gamma" : Outport
  " 1+nu.Phi.G.Phi" : Outport  Port=2
  wires:
  "gamma "/1 -> Scope3/1, [gamma], " gamma"/1
  " "/1 -> Switch/1
  vDv/1(Out1) -> Scope/1, Switch/2
  Phi_f/1 -> Gamma_dot/1(Phi_f)
  Gamma_dot/1(gamma_dot) -> Scope2/1, InitializationDelay/1(u)
  [gamma] -> Gamma_dot/2(Gamma)
  Gamma_dot/2(" 1+nu.Phi.G.Phi") -> " 1+nu.Phi.G.Phi"/1
  Product/1 -> "gamma "/1, Switch/3, vDv/1(In1)
  Switch/1 -> Scope1/1
  InitializationDelay/1(y) -> Product/1
  Adapt/1 -> Product/2

== system IARC_Nonlinear_Sensors/ARC Controller/Position Control/X control/Adaptation Law_X/Integral Type Adaptation Law Discontinuous Projection1/InitializationDelay ==
  u : Inport
  Clock : Clock
  Compare To Constant2 : simulink/Logic and Bit Operations/Compare To Constant  relop=>=  const=t0  OutDataTypeStr=boolean
  Data Type Conversion : DataTypeConversion
  Product : Product
  y : Outport
  wires:
  u/1 -> Product/1
  Compare To Constant2/1 -> Data Type Conversion/1
  Clock/1 -> Compare To Constant2/1
  Data Type Conversion/1 -> Product/2
  Product/1 -> y/1

== system IARC_Nonlinear_Sensors/ARC Controller/Position Control/Y control/Adaptation Law_Y/IARC, Physical Model Based Parameter Estimation (69)_X/Discontinuous_Proj_(49) ==
  Theta_dot : Inport
  Adapt : Inport  Port=2
  Integrator1 : Integrator  InitialCondition=theta_0  UpperSaturationLimit=theta_max  LowerSaturationLimit=theta_min
  Integrator2 : Integrator  Commented=on  InitialCondition=theta_0  LimitOutput=on  UpperSaturationLimit=theta_max  LowerSaturationLimit=theta_min
  Product : Product
  Saturation : Saturate  UpperLimit=Theta_dot_M  LowerLimit=-Theta_dot_M
  Theta : Outport
  wires:
  Integrator1/1 -> Theta/1
  Product/1 -> Saturation/1
  Saturation/1 -> Integrator1/1
  Adapt/1 -> Product/2
  Theta_dot/1 -> Product/1

== system IARC_Nonlinear_Sensors/ARC Controller/Position Control/Y control/Adaptation Law_Y/IARC, Physical Model Based Parameter Estimation (69)_X/Epsilon ==
  f(x)_f_dot : Inport
  Phi_f : Inport  Port=2
  Theta_hat : Inport  Port=3
  Math Function : Math  Operator=transpose  SaturateOnIntegerOverflow=on
  Mux1 : Mux  Inputs=3
  Product1 : Product  Multiplication=Matrix(*)
  Subtract : Sum  Inputs=+-
  "epsilon  " : Scope
  Epsilon : Outport
  wires:
  f(x)_f_dot/1 -> Mux1/2, Subtract/1  "Yp"
  Product1/1 -> Mux1/3, Subtract/2  "Yp_hat"
  Phi_f/1 -> Math Function/1
  Theta_hat/1 -> Product1/2
  Math Function/1 -> Product1/1
  Subtract/1 -> Mux1/1, Epsilon/1
  Mux1/1 -> "epsilon  "/1

== system IARC_Nonlinear_Sensors/ARC Controller/Position Control/Y control/Adaptation Law_Y/IARC, Physical Model Based Parameter Estimation (69)_X/Filter ==
  f(x) : Inport
  "Phi " : Inport  Port=2
  Mux1 : Mux  Commented=on  Inputs=2
  Mux2 : Mux  Commented=on  Inputs=2
  filter : TransferFcn  Denominator=[Tau 1]
  "filter " : TransferFcn  Denominator=[Tau 1]
  gamma : Scope  Commented=on
  gamma1 : Scope  Commented=on
  f(x)_f : Outport
  Phi_f : Outport  Port=2
  wires:
  f(x)/1 -> "filter "/1, Mux1/1
  Mux1/1 -> gamma/1
  Mux2/1 -> gamma1/1
  "Phi "/1 -> filter/1, Mux2/1
  "filter "/1 -> f(x)_f/1, Mux1/2
  filter/1 -> Mux2/2, Phi_f/1

== system IARC_Nonlinear_Sensors/ARC Controller/Position Control/Y control/Adaptation Law_Y/IARC, Physical Model Based Parameter Estimation (69)_X/Gamma ==
  Phi_f : Inport
  Adapt : Inport  Port=2
  " " : Constant  Value=diag(0,0)
  Gamma_dot : Subsystem
  InitializationDelay : Subsystem  AncestorBlock=UAV_Control/InitializationDelay  mask(InitializationDelay){t0=t1}
      mask prompts: t0 "Initialization delay:"
      mask help: Applays a delay before passing the first signal.
      mask Help: Applays a delay (t0) before passing the first signal
      mask Display:
      | port_label('input',1,'u','texmode','on')
      | port_label('output',1,'y','texmode','on')
  Product : Product
  Scope{,1..3} (4 alike) : Scope  Commented=on
  Switch : Switch  Criteria=u2 > Threshold
  "gamma " : Integrator  InitialCondition=gamma0  LimitOutput=on  UpperSaturationLimit=Rho_M  LowerSaturationLimit=Rho_L
  vDv : Subsystem
  " gamma" : Outport
  " 1+nu.Phi.G.Phi" : Outport  Port=2
  wires:
  "gamma "/1 -> Scope3/1, [gamma], " gamma"/1
  " "/1 -> Switch/1
  vDv/1(Out1) -> Scope/1, Switch/2
  Phi_f/1 -> Gamma_dot/1(Phi_f)
  Gamma_dot/1(gamma_dot) -> Scope2/1, InitializationDelay/1(u)
  [gamma] -> Gamma_dot/2(Gamma)
  Gamma_dot/2(" 1+nu.Phi.G.Phi") -> " 1+nu.Phi.G.Phi"/1
  Product/1 -> "gamma "/1, Switch/3, vDv/1(In1)
  Switch/1 -> Scope1/1
  InitializationDelay/1(y) -> Product/1
  Adapt/1 -> Product/2

== system IARC_Nonlinear_Sensors/ARC Controller/Position Control/Y control/Adaptation Law_Y/Integral Type Adaptation Law Discontinuous Projection1/InitializationDelay ==
  u : Inport
  Clock : Clock
  Compare To Constant2 : simulink/Logic and Bit Operations/Compare To Constant  relop=>=  const=t0  OutDataTypeStr=boolean
  Data Type Conversion : DataTypeConversion
  Product : Product
  y : Outport
  wires:
  u/1 -> Product/1
  Compare To Constant2/1 -> Data Type Conversion/1
  Clock/1 -> Compare To Constant2/1
  Data Type Conversion/1 -> Product/2
  Product/1 -> y/1

== system IARC_Nonlinear_Sensors/ARC Controller/Position Control/Z control/Estimate theta = K//m/IARC, Physical Model Based Parameter Estimation (69)/Discontinuous_Proj_(49) ==
  Theta_dot : Inport
  Adapt : Inport  Port=2
  Integrator2 : Integrator  InitialCondition=theta_0  LimitOutput=on  UpperSaturationLimit=theta_max  LowerSaturationLimit=theta_min
  Product : Product
  Saturation : Saturate  UpperLimit=Theta_dot_M  LowerLimit=-Theta_dot_M
  theta dot : Scope  Commented=on
  Theta : Outport
  wires:
  Theta_dot/1 -> Product/1
  Adapt/1 -> Product/2
  Integrator2/1 -> Theta/1
  Product/1 -> Saturation/1
  Saturation/1 -> theta dot/1, Integrator2/1

== system IARC_Nonlinear_Sensors/ARC Controller/Position Control/Z control/Estimate theta = K//m/IARC, Physical Model Based Parameter Estimation (69)/Epsilon ==
  y_f : Inport
  Phi_f : Inport  Port=2
  Theta_hat : Inport  Port=3
  Math Function : Math  Operator=transpose  SaturateOnIntegerOverflow=on
  Mux3 : Mux  Inputs=3
  Product1 : Product  Multiplication=Matrix(*)
  Subtract : Sum  Inputs=+-
  epsilon  2 : Scope
  Epsilon : Outport
  wires:
  y_f/1 -> Mux3/1, Subtract/1  "Yp"
  Subtract/1 -> Mux3/3, Epsilon/1
  Product1/1 -> Mux3/2, Subtract/2  "Yp_hat"
  Phi_f/1 -> Math Function/1
  Theta_hat/1 -> Product1/2
  Math Function/1 -> Product1/1
  Mux3/1 -> epsilon  2/1

== system IARC_Nonlinear_Sensors/ARC Controller/Position Control/Z control/Estimate theta = K//m/IARC, Physical Model Based Parameter Estimation (69)/Filter ==
  y : Inport
  "Phi " : Inport  Port=2
  Demux : Demux  Outputs=2
  Mux1 : Mux  Commented=on  Inputs=2
  Mux2 : Mux  Commented=on  Inputs=2
  Mux3 : Mux  Inputs=2
  filter : TransferFcn  Denominator=[Tau 1]
  "filter " : TransferFcn  Denominator=[Tau 1]
  gamma : Scope  Commented=on
  gamma1 : Scope  Commented=on
  y_f : Outport
  Phi_f : Outport  Port=2
  wires:
  filter/1 -> Mux3/1, Mux2/2
  "filter "/1 -> y_f/1, Mux1/2
  y/1 -> Mux1/1, "filter "/1
  Mux1/1 -> gamma/1
  Demux/1 -> filter/1, Mux2/1
  Mux2/1 -> gamma1/1
  "Phi "/1 -> Demux/1
  Mux3/1 -> Phi_f/1
  Demux/2 -> Mux3/2

== system IARC_Nonlinear_Sensors/ARC Controller/Position Control/Z control/Estimate theta = K//m/IARC, Physical Model Based Parameter Estimation (69)/Gamma ==
  Phi_f : Inport
  Adapt : Inport  Port=2
  " " : Constant  Value=0
  Gamma_dot : Subsystem
  InitializationDelay : Subsystem  AncestorBlock=UAV_Control/InitializationDelay  mask(InitializationDelay){t0=t1}
      mask prompts: t0 "Initialization delay:"
      mask help: Applays a delay before passing the first signal.
      mask Help: Applays a delay (t0) before passing the first signal
      mask Display:
      | port_label('input',1,'u','texmode','on')
      | port_label('output',1,'y','texmode','on')
  Product : Product
  Scope{,1..3} (4 alike) : Scope  Commented=on
  Switch : Switch  Criteria=u2 > Threshold
  "gamma " : Integrator  InitialCondition=gamma0  LimitOutput=on  UpperSaturationLimit=Rho_M  LowerSaturationLimit=Rho_L
  vDv : Subsystem
  " gamma" : Outport
  " 1+nu.Phi.G.Phi" : Outport  Port=2
  wires:
  InitializationDelay/1(y) -> Product/1
  Adapt/1 -> Product/2
  "gamma "/1 -> Scope3/1, [gamma], " gamma"/1
  " "/1 -> Switch/1
  vDv/1(Out1) -> Scope/1, Switch/2
  Phi_f/1 -> Gamma_dot/1(Phi_f)
  Gamma_dot/1(gamma_dot) -> Scope2/1, InitializationDelay/1(u)
  [gamma] -> Gamma_dot/2(Gamma)
  Gamma_dot/2(" 1+nu.Phi.G.Phi") -> " 1+nu.Phi.G.Phi"/1
  Product/1 -> vDv/1(In1), "gamma "/1, Switch/3
  Switch/1 -> Scope1/1

== system IARC_Nonlinear_Sensors/ARC Controller/Position Control/Z control/Estimate theta = K//m/Integral Type Adaptation Law Discontinuous Projection/InitializationDelay ==
  u : Inport
  Clock : Clock
  Compare To Constant2 : simulink/Logic and Bit Operations/Compare To Constant  relop=>=  const=t0  OutDataTypeStr=boolean
  Data Type Conversion : DataTypeConversion
  Product : Product
  y : Outport
  wires:
  u/1 -> Product/1
  Compare To Constant2/1 -> Data Type Conversion/1
  Clock/1 -> Compare To Constant2/1
  Data Type Conversion/1 -> Product/2
  Product/1 -> y/1

== system IARC_Nonlinear_Sensors/Sensors and Filters/Data processing/Estimate Position/Signal Conditioning - Sonar/Sampler/Triggered Subsystem ==
  In1 : Inport
  Trigger : TriggerPort  VariantControl=(inherit)
  Out1 : Outport
  wires:
  In1/1 -> Out1/1

== system IARC_Nonlinear_Sensors/ARC Controller/Attitutde Control/Yaw control/Subsystem/IARC, Physical Model Based Parameter Estimation (69)_Yaw/Gamma/Gamma_dot ==
  note: D.Gamma=mu1.G-mu2.G.P.P.G
      |
      | Normalized:
      | D.Gamma=alpha.G-(G.P.P.G)/(1+nu.P.GP)
  Phi_f : Inport
  Gamma : Inport  Port=2
  " " : Gain  Gain=mu2
  "  (Normalized)" : Gain  Gain=nu
  Add : Sum  Inputs=+-
  Add1 : Sum
  Add2 : Sum  Inputs=+-
  Constant : Constant
  Constant4 : Constant  Value=Norm_ON
  Divide : Product  Inputs=*/
  G.P.P.G : Product  Inputs=4  Multiplication=Matrix(*)
  Gamma1 : InportShadow  Port=2
  Gamma2 : InportShadow  Port=2
  P.G.P : Product  Inputs=3  Multiplication=Matrix(*)
  Switch2 : Switch  Threshold=0.5
  Transpose1 : Math  Operator=transpose  SaturateOnIntegerOverflow=on
  "forgetting factor " : Gain  Gain=mu1
  forgetting factor (Normalized) : Gain  Gain=alpha
  gamma_dot : Outport
  " 1+nu.Phi.G.Phi" : Outport  Port=2
  wires:
  "  (Normalized)"/1 -> Add1/2
  Phi_f/1 -> P.G.P/3, Transpose1/1, G.P.P.G/2
  Transpose1/1 -> P.G.P/1, G.P.P.G/3
  Gamma/1 -> G.P.P.G/1, P.G.P/2, G.P.P.G/4
  "forgetting factor "/1 -> Add/1
  G.P.P.G/1 -> " "/1, Divide/1
  Constant/1 -> Add1/1
  P.G.P/1 -> "  (Normalized)"/1
  Add1/1 -> Divide/2, " 1+nu.Phi.G.Phi"/1
  Gamma2/1 -> forgetting factor (Normalized)/1
  Add2/1 -> Switch2/1
  Constant4/1 -> Switch2/2
  Add/1 -> Switch2/3
  Switch2/1 -> gamma_dot/1
  Divide/1 -> Add2/2
  forgetting factor (Normalized)/1 -> Add2/1
  " "/1 -> Add/2
  Gamma1/1 -> "forgetting factor "/1

== system IARC_Nonlinear_Sensors/ARC Controller/Attitutde Control/Yaw control/Subsystem/IARC, Physical Model Based Parameter Estimation (69)_Yaw/Gamma/InitializationDelay ==
  u : Inport
  Clock : Clock
  Compare To Constant2 : simulink/Logic and Bit Operations/Compare To Constant  relop=>=  const=t0  OutDataTypeStr=boolean
  Data Type Conversion : DataTypeConversion
  Product : Product
  y : Outport
  wires:
  u/1 -> Product/1
  Compare To Constant2/1 -> Data Type Conversion/1
  Clock/1 -> Compare To Constant2/1
  Data Type Conversion/1 -> Product/2
  Product/1 -> y/1

== system IARC_Nonlinear_Sensors/ARC Controller/Attitutde Control/Yaw control/Subsystem/IARC, Physical Model Based Parameter Estimation (69)_Yaw/Gamma/vDv ==
  In1 : Inport
  Product2 : Product  Inputs=3  Multiplication=Matrix(*)
  Transpose2 : Math  Operator=transpose  SaturateOnIntegerOverflow=on
  eigenvector of Gamm_max : Constant  Value=v
  Out1 : Outport
  wires:
  Transpose2/1 -> Product2/1
  In1/1 -> Product2/2
  eigenvector of Gamm_max/1 -> Transpose2/1, Product2/3
  Product2/1 -> Out1/1

== system IARC_Nonlinear_Sensors/ARC Controller/Attitutde Control/pitch control/Adaptation Law_X/IARC, Physical Model Based Parameter Estimation (69)_pitch (theta)/Gamma/Gamma_dot ==
  note: D.Gamma=mu1.G-mu2.G.P.P.G
      |
      | Normalized:
      | D.Gamma=alpha.G-(G.P.P.G)/(1+nu.P.GP)
  Phi_f : Inport
  Gamma : Inport  Port=2
  " " : Gain  Gain=mu2
  "  (Normalized)" : Gain  Gain=nu
  Add : Sum  Inputs=+-
  Add1 : Sum
  Add2 : Sum  Inputs=+-
  Constant : Constant
  Constant4 : Constant  Value=Norm_ON
  Divide : Product  Inputs=*/
  G.P.P.G : Product  Inputs=4  Multiplication=Matrix(*)
  Gamma1 : InportShadow  Port=2
  Gamma2 : InportShadow  Port=2
  P.G.P : Product  Inputs=3  Multiplication=Matrix(*)
  Switch2 : Switch  Threshold=0.5
  Transpose1 : Math  Operator=transpose  SaturateOnIntegerOverflow=on
  "forgetting factor " : Gain  Gain=mu1
  forgetting factor (Normalized) : Gain  Gain=alpha
  gamma_dot : Outport
  " 1+nu.Phi.G.Phi" : Outport  Port=2
  wires:
  "  (Normalized)"/1 -> Add1/2
  Phi_f/1 -> P.G.P/3, Transpose1/1, G.P.P.G/2
  Transpose1/1 -> P.G.P/1, G.P.P.G/3
  Gamma/1 -> G.P.P.G/1, P.G.P/2, G.P.P.G/4
  "forgetting factor "/1 -> Add/1
  G.P.P.G/1 -> " "/1, Divide/1
  Constant/1 -> Add1/1
  P.G.P/1 -> "  (Normalized)"/1
  Add1/1 -> Divide/2, " 1+nu.Phi.G.Phi"/1
  Gamma2/1 -> forgetting factor (Normalized)/1
  Add2/1 -> Switch2/1
  Constant4/1 -> Switch2/2
  Add/1 -> Switch2/3
  Switch2/1 -> gamma_dot/1
  Divide/1 -> Add2/2
  forgetting factor (Normalized)/1 -> Add2/1
  " "/1 -> Add/2
  Gamma1/1 -> "forgetting factor "/1
